simulink model "MTE360prelab2simulink"  (R2024a)
settings: Solver=VariableStepAuto  StartTime=0.0  StopTime=10  RelTol=1e-3
undefined symbols (not defined in the file): Alpha, b, Kd, Ki, Kp, m
settings Model: Creator=j2668li  LastModifiedBy=d49gupta

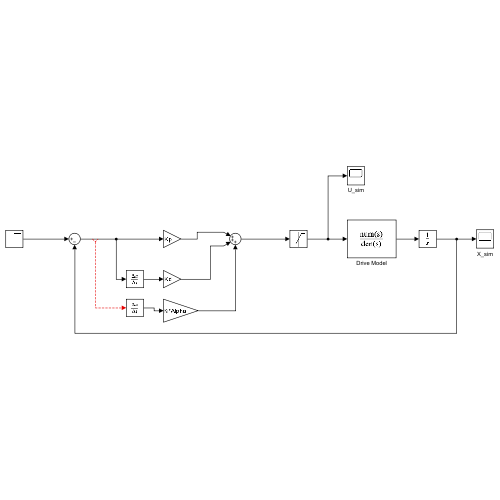
[thumbnail: Simulink's stored preview of the top-level diagram]
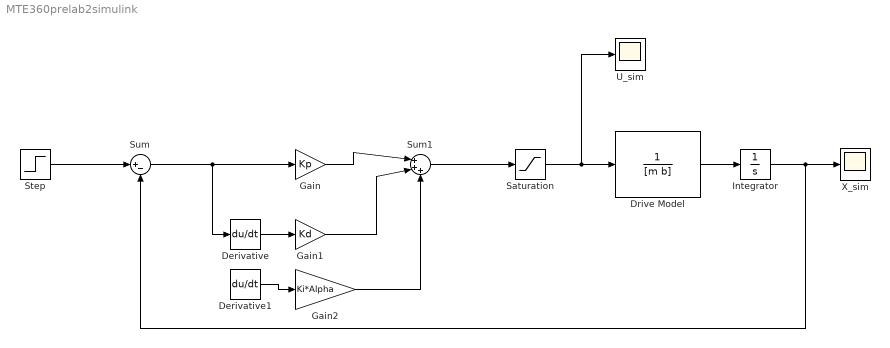
== system MTE360prelab2simulink ==
  Derivative : Derivative
  Derivative1 : Derivative
  Drive Model : TransferFcn  Denominator=[m b]
  Gain : Gain  Gain=Kp
  Gain1 : Gain  Gain=Kd
  Gain2 : Gain  Gain=Ki*Alpha
  Integrator : Integrator
  Saturation : Saturate
  Step : Step  After=10  SampleTime=0
  Sum : Sum  Inputs=|+-
  Sum1 : Sum  Inputs=|+++
  U_sim : Scope
  X_sim : Scope
  wires:
  Step/1 -> Sum/1
  Sum/1 -> Derivative/1, Gain/1
  Derivative/1 -> Gain1/1
  Gain/1 -> Sum1/1
  Sum1/1 -> Saturation/1
  Saturation/1 -> U_sim/1, Drive Model/1
  Drive Model/1 -> Integrator/1
  Integrator/1 -> Sum/2, X_sim/1
  Gain1/1 -> Sum1/2
  Derivative1/1 -> Gain2/1
  ? -> Derivative1/1
  Gain2/1 -> Sum1/3
